simulink model "DrocketDynamic"  (R2021a)
settings: Solver=VariableStepAuto  StartTime=0.0  StopTime=44  RelTol=1e-3
values from neighbouring files (symbols this model uses):
  Cd = 0.5    [1DrocketDynamics.mat]
  g = 9.81    [1DrocketDynamics.mat]
  m = 30    [1DrocketDynamics.mat]
  rho = 1.225    [1DrocketDynamics.mat]
  S = 0.0113097335529    [1DrocketDynamics.mat]
  Thrust_Vector = [1500 1500 1500 1500 1500]    [1DrocketDynamics.mat]
undefined symbols (not defined in the file or in its folder): magnitude
libraries: simulink x2
settings Model: Creator=kadir  LastModifiedBy=kadir

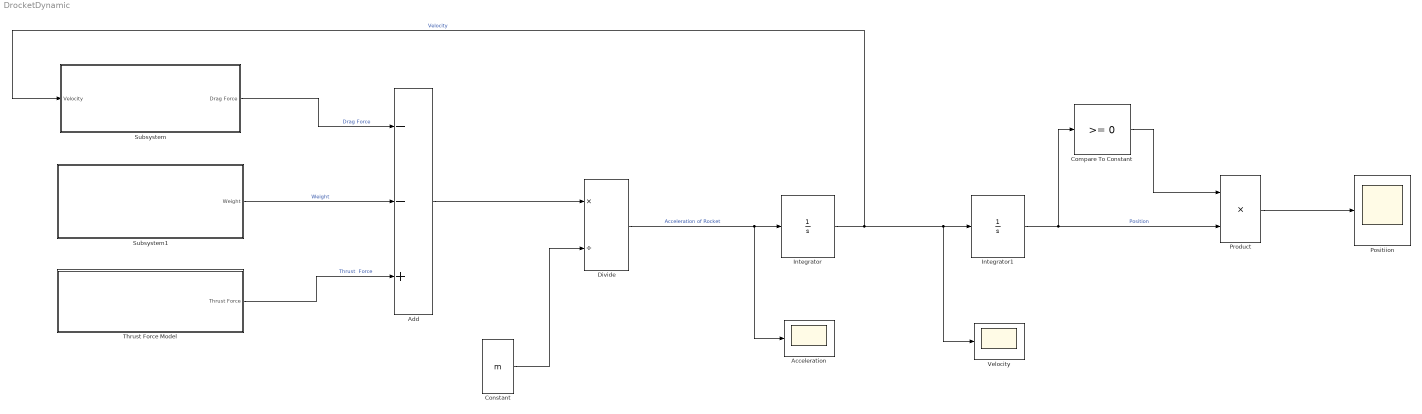
== system DrocketDynamic ==
  Acceleration : Scope
  Add : Sum  Inputs=--+
  Compare To Constant : simulink/Logic and Bit Operations/Compare To Constant  relop=>=  const=0  OutDataTypeStr=boolean
  Constant : Constant  Value=m
  Divide : Product  Inputs=*/
  Integrator : Integrator
  Integrator1 : Integrator
  Positiion : Scope
  Product : Product
  Subsystem : Subsystem
  Subsystem1 : Subsystem
  Thrust Force Model : Subsystem
  Velocity : Scope
  wires:
  Integrator/1 -> Subsystem/1(Velocity), Velocity/1, Integrator1/1  "Velocity"
  Subsystem/1(Drag Force) -> Add/1  "Drag Force"
  Subsystem1/1(Weight) -> Add/2  "Weight"
  Thrust Force Model/1(Thrust Force) -> Add/3  "Thrust  Force"
  Add/1 -> Divide/1
  Constant/1 -> Divide/2
  Divide/1 -> Acceleration/1, Integrator/1  "Acceleration of Rocket"
  Integrator1/1 -> Compare To Constant/1, Product/2  "Position"
  Compare To Constant/1 -> Product/1
  Product/1 -> Positiion/1

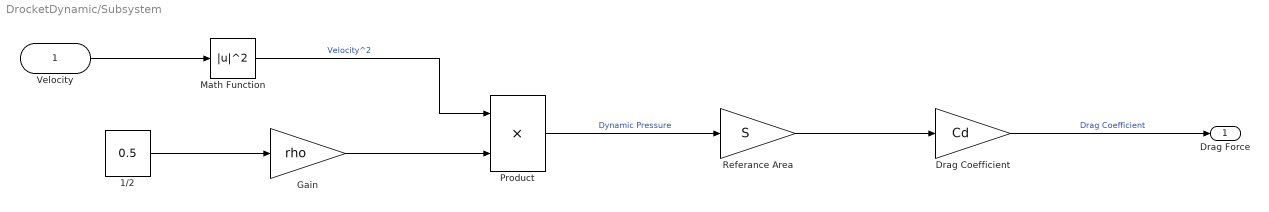
== system DrocketDynamic/Subsystem ==
  Velocity : Inport
  1/2 : Constant  Value=0.5
  Drag Coefficient : Gain  Gain=Cd
  Gain : Gain  Gain=rho
  Math Function : Math  Operator=magnitude^2  SaturateOnIntegerOverflow=on
  Product : Product
  Referance Area : Gain  Gain=S
  Drag Force : Outport
  wires:
  Drag Coefficient/1 -> Drag Force/1  "Drag Coefficient"
  1/2/1 -> Gain/1
  Gain/1 -> Product/2
  Referance Area/1 -> Drag Coefficient/1
  Math Function/1 -> Product/1  "Velocity^2"
  Velocity/1 -> Math Function/1
  Product/1 -> Referance Area/1  "Dynamic Pressure"

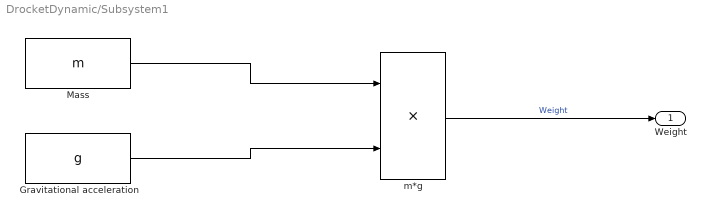
== system DrocketDynamic/Subsystem1 ==
  Gravitational acceleration : Constant  Value=g
  Mass : Constant  Value=m
  m*g : Product
  Weight : Outport
  wires:
  Gravitational acceleration/1 -> m*g/2
  Mass/1 -> m*g/1
  m*g/1 -> Weight/1  "Weight"

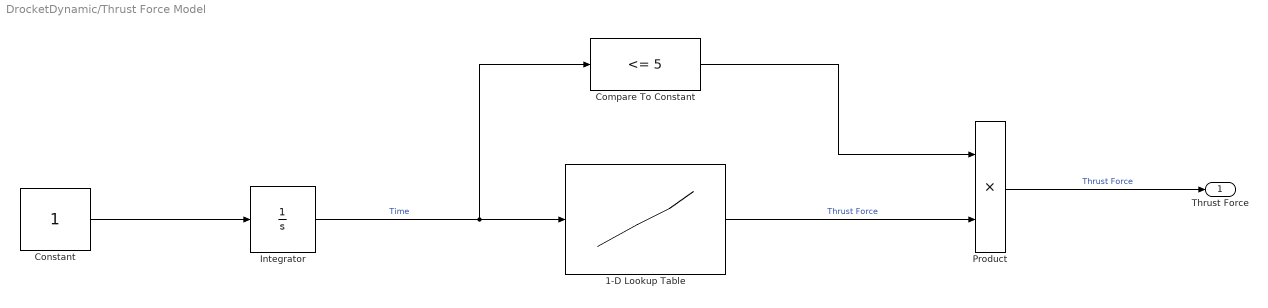
== system DrocketDynamic/Thrust Force Model ==
  1-D Lookup Table : Lookup_n-D  NumberOfTableDimensions=1  BreakpointsForDimension1=[1:5]  Table=Thrust_Vector  InternalRulePriority=Speed  RndMeth=Simplest  InputSameDT=on
  Compare To Constant : simulink/Logic and Bit Operations/Compare To Constant  relop=<=  const=5  OutDataTypeStr=boolean
  Constant : Constant
  Integrator : Integrator
  Product : Product
  Thrust Force : Outport
  wires:
  Integrator/1 -> Compare To Constant/1, 1-D Lookup Table/1  "Time"
  1-D Lookup Table/1 -> Product/2  "Thrust Force"
  Constant/1 -> Integrator/1
  Compare To Constant/1 -> Product/1
  Product/1 -> Thrust Force/1  "Thrust Force"
